simulink model "lab3_otau"  (R2014a)
settings: Solver=ode45  StartTime=0.0  StopTime=100.0  RelTol=1e-3
settings Model: Creator=user  LastModifiedBy=user

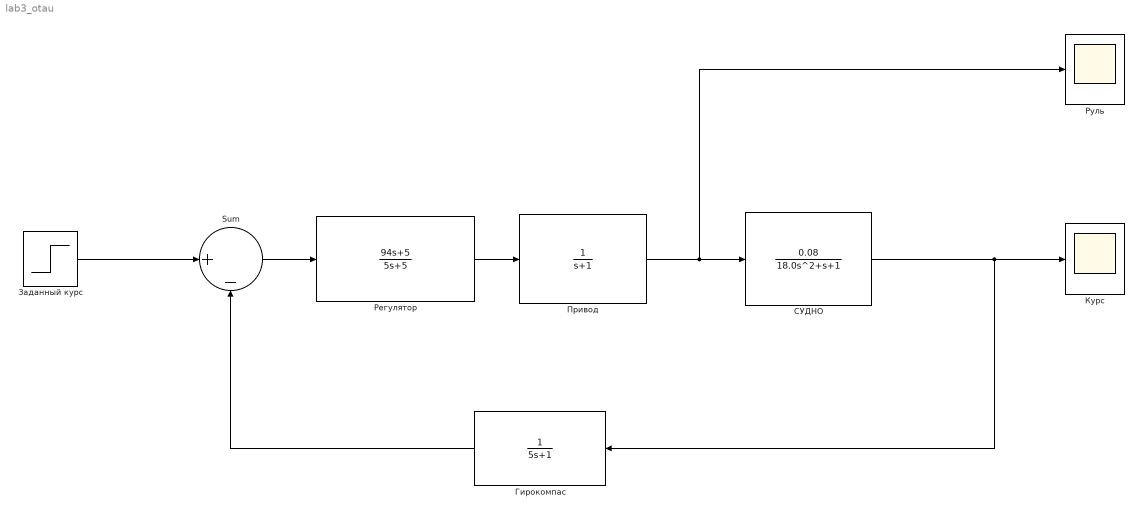
== system lab3_otau ==
  "\tСУДНО" : TransferFcn  Numerator=[0.08]  Denominator=[18.0 1 1]
  Sum : Sum  Inputs=|+-
  Гирокомпас : TransferFcn  Denominator=[5 1]
  Заданный курс : Step  Time=0  After=10  SampleTime=0
  Курс : Scope
  Привод : TransferFcn  Denominator=[1 1]
  Регулятор : TransferFcn  Numerator=[94 5]  Denominator=[5 5]
  Руль : Scope
  wires:
  Заданный курс/1 -> Sum/1
  Sum/1 -> Регулятор/1
  Регулятор/1 -> Привод/1
  "\tСУДНО"/1 -> Гирокомпас/1, Курс/1
  Привод/1 -> Руль/1, "\tСУДНО"/1
  Гирокомпас/1 -> Sum/2
